simulink model "simpong3"  (R2012b)
settings: Solver=ode1  StartTime=0.0  StopTime=inf  FixedStep=1  RelTol=1e-3
libraries: simulink x1
settings Model: Creator=caster  LastModifiedBy=caster

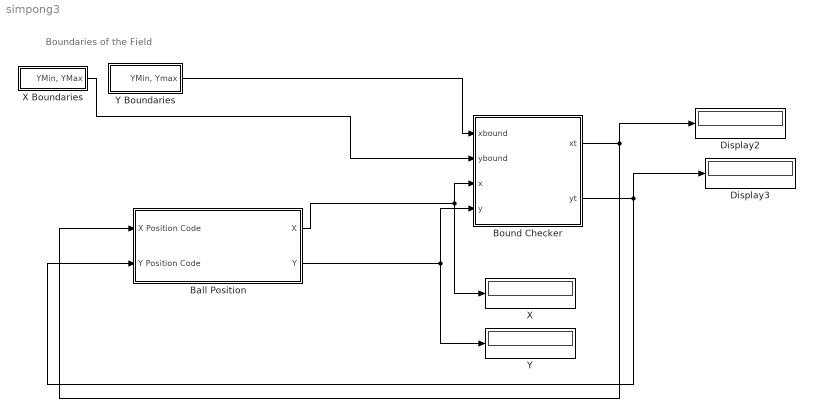
== system simpong3 ==
  note: Boundaries of the Field
  Ball Position : Subsystem
  Bound Checker : MATLAB Function  TreatAsAtomicUnit=on
  Display2 : Display
  Display3 : Display
  X : Display
  X Boundaries : Subsystem
  Y : Display
  Y Boundaries : Subsystem
  wires:
  Bound Checker/1(xt) -> Ball Position/1(X Position Code), Display2/1
  Bound Checker/2(yt) -> Ball Position/2(Y Position Code), Display3/1
  X Boundaries/1("YMin, YMax") -> Bound Checker/2(ybound)
  Y Boundaries/1("YMin, Ymax") -> Bound Checker/1(xbound)
  Ball Position/1(X) -> X/1, Bound Checker/3(x)
  Ball Position/2(Y) -> Y/1, Bound Checker/4(y)

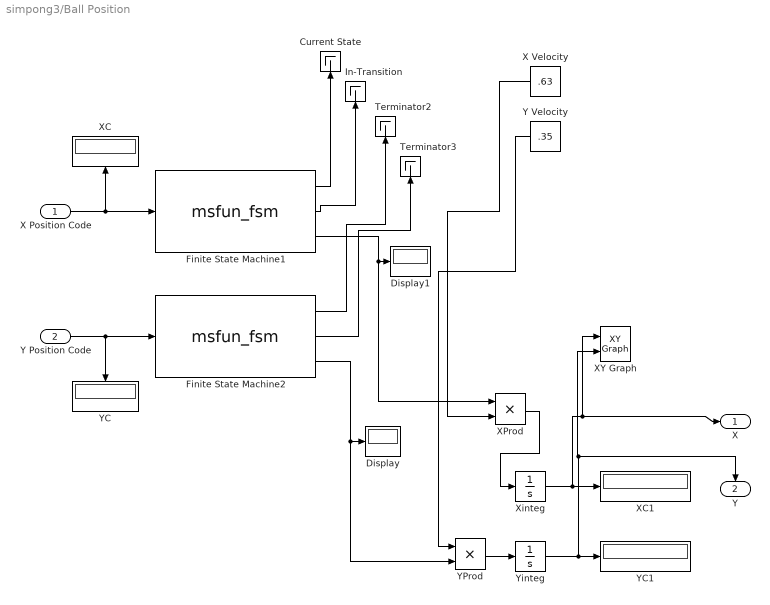
== system simpong3/Ball Position ==
  X Position Code : Inport
  Y Position Code : Inport  Port=2
  Current State : Terminator
  Display : Display
  Display1 : Display
  Finite State Machine1 : M-S-Function  FunctionName=msfun_fsm  Parameters=nsts, outs, initState, ansts, irp, errortrans  mask(Finite State Machine){initState=1, outs=[[1,1];[-1,-1]], nsts=[[1,5,-1];[1,-5,-1];[-1,5,1];[-1,-5,1]], errortrans=[], ansts=[], irp=on}
      mask prompts: initState "Initial State:"; outs "Output Functions"; nsts "Next State Transitions"; errortrans "Error Transitions"; ansts "Absolute Next-State Transitions"; irp "Ignore Repeated Inputs?"
      mask help: This block allows one to enter in various parameters of a finite state machine.
      mask Display:
      | port_label('input',1,'Input Signals');
      | port_label('output',1,'Current State');
      | port_label('output',2,'In-transition');
      | port_label('output',3,'Output Signal');
  Finite State Machine2 : M-S-Function  FunctionName=msfun_fsm  Parameters=nsts, outs, initState, ansts, irp  mask(Finite State Machine){initState=1, nsts=[[1,5,-1];[1,-5,-1];[-1,5,1];[-1,-5,1]], outs=[[1,1];[-1,-1]], ansts=[], irp=on}
      mask prompts: initState "Initial State:"; nsts "Next State Transitions"; outs "Output Functions"; ansts "Absolute Next-State Transitions"; irp "Ignore Repeated Inputs?"
      mask help: This block allows one to enter in various parameters of a finite state machine.
      mask Display:
      | port_label('input',1,'Input Signals');
      | port_label('output',1,'Current State');
      | port_label('output',2,'In-transition');
      | port_label('output',3,'Output Signal');
  In-Transition : Terminator
  Terminator2 : Terminator
  Terminator3 : Terminator
  X Velocity : Constant  Value=.63
  XC : Display
  XC1 : Display
  XProd : Product  RndMeth=Zero
  XY Graph : simulink/Sinks/XY Graph  xmin=-10  xmax=10  ymin=-10  ymax=10  st=-1
  Xinteg : Integrator
  Y Velocity : Constant  Value=.35
  YC : Display
  YC1 : Display
  YProd : Product  RndMeth=Zero
  Yinteg : Integrator
  X : Outport
  Y : Outport  Port=2
  wires:
  X Velocity/1 -> XProd/2
  Xinteg/1 -> XC1/1, X/1, XY Graph/1
  Y Velocity/1 -> YProd/1
  Yinteg/1 -> Y/1, XY Graph/2, YC1/1
  X Position Code/1 -> Finite State Machine1/1, XC/1
  Y Position Code/1 -> Finite State Machine2/1, YC/1
  Finite State Machine2/3 -> YProd/2, Display/1
  XProd/1 -> Xinteg/1
  YProd/1 -> Yinteg/1
  Finite State Machine1/3 -> Display1/1, XProd/1
  Finite State Machine1/1 -> Current State/1
  Finite State Machine1/2 -> In-Transition/1
  Finite State Machine2/1 -> Terminator2/1
  Finite State Machine2/2 -> Terminator3/1

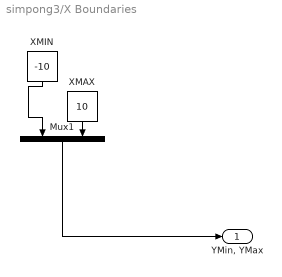
== system simpong3/X Boundaries ==
  Mux1 : Mux  Inputs=2
  XMAX : Constant  Value=10
  XMIN : Constant  Value=-10
  "YMin, YMax" : Outport
  wires:
  XMAX/1 -> Mux1/2
  Mux1/1 -> "YMin, YMax"/1
  XMIN/1 -> Mux1/1

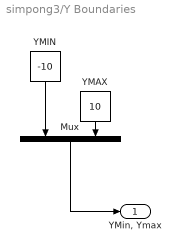
== system simpong3/Y Boundaries ==
  Mux : Mux  Inputs=2
  YMAX : Constant  Value=10
  YMIN : Constant  Value=-10
  "YMin, Ymax" : Outport
  wires:
  YMIN/1 -> Mux/1
  YMAX/1 -> Mux/2
  Mux/1 -> "YMin, Ymax"/1

== matlab function simpong3/Bound Checker ==
  data: xbound input; ybound input; x input; y input; xt output; yt output
function [xt,yt] = fcn(xbound,ybound,x,y)

    if x > xbound(2)
        xt = 5;
    elseif x < xbound(1)
        xt = -5;
    else
        xt = 0;
    end
    
    if y > ybound(2)
        yt = 5;
    elseif y < ybound(1)
        yt = -5;
    else
        yt = 0;
    end
    
end
